simulink model "lab4_1 (1)"  (R2018b)
settings: Solver=ode4  StartTime=0.0  StopTime=10  FixedStep=0.01  RelTol=1e-3
values from neighbouring files (symbols this model uses):
  A = Rs*(Ps^(-1))    [lab4m (1).m]
  B = [ 0; 0]    [lab4m (1).m]
  C = [ 1 0 ; 0 1 ]    [lab4m (1).m]
  D = [ 0 ; 0 ]    [lab4m (1).m]
settings Model: Creator=Jakub  LastModifiedBy=PanLapek
settings SFSimCC: SimUseLocalCustomCode=off
settings RTWCC: RTWUseLocalCustomCode=off

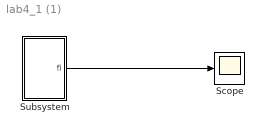
== system lab4_1 (1) ==
  Scope : Scope
  Subsystem : Subsystem  mask{m=2, l=1, k=2, g=9.81, fi0=90}
      mask prompts: m "Masa"; l "Dlugosc"; fi0 "fi"
  wires:
  Subsystem/1("fi ") -> Scope/1

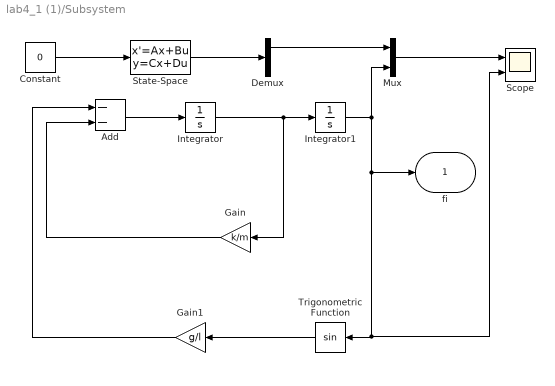
== system lab4_1 (1)/Subsystem ==
  Add : Sum  Inputs=--
  Constant : Constant  Value=0
  Demux : Demux  Outputs=2
  Gain : Gain  Gain=k/m
  Gain1 : Gain  Gain=g/l
  Integrator : Integrator
  Integrator1 : Integrator  InitialCondition=(fi0*pi)/180
  Mux : Mux  Inputs=2
  Scope : Scope  NumInputPorts=2
  State-Space : StateSpace  A=A  B=B  C=C  D=D  InitialCondition=[pi/2 0]
  Trigonometric Function : Trigonometry
  "fi " : Outport
  wires:
  Gain1/1 -> Add/1
  Gain/1 -> Add/2
  Add/1 -> Integrator/1
  Integrator1/1 -> Mux/2, Scope/2, Trigonometric Function/1, "fi "/1
  Trigonometric Function/1 -> Gain1/1
  Constant/1 -> State-Space/1
  Integrator/1 -> Gain/1, Integrator1/1
  State-Space/1 -> Demux/1
  Demux/1 -> Mux/1
  Mux/1 -> Scope/1
